simulink model "explicitCompFilter_uORB"  (R2024b)
settings: Solver=FixedStepAuto  StartTime=0.0  StopTime=35  FixedStep=0.005  RelTol=1e-3  EnableMultiTasking=on
PreLoadFcn:
  | %b_prev = Simulink.Signal;
  | %q_prev = Simulink.Signal;
  | 
  | %b_prev.InitialValue = '[0; 0; 0]';
  | %q_prev.InitialValue = '[0; 0; 0; 0]';
InitFcn:
  | %g_or = [0;0;-9.81];
  | %m_or = [27.5550; 2.4169; 16.0849];
  | gyroBias = [1; 1; 0.5];
  | 
  | %IF USING BUILT-IN UAV ANIMATION, uncomment below
  | 
  | %CLEAR UAV ANIMATIONS
  | %figHandles = findall(groot, 'Type', 'figure');
  | 
  | %for i=1:size(figHandles)
  | %    figObj = figHandles(i);
  | %    figName = figObj.Name;
  | %   if contains(figName, 'UAV Animation');
  | %        delete(figObj);
  | %    end
  | %end
undefined symbols (not defined in the file): g
libraries: robotcorelib x3, simulink_extras x3, px4Sensorslib x2, simulink x1, matrix_library x1, vrlib x1, px4uORBlib x1
(part 2 of 3)

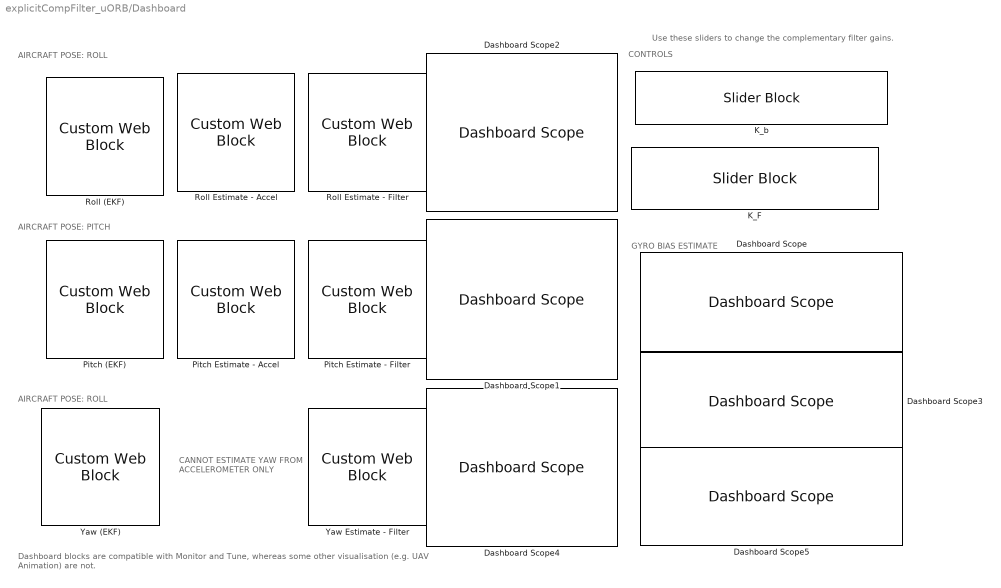
== system explicitCompFilter_uORB/Dashboard ==
  note: Dashboard blocks are compatible with Monitor and Tune, whereas some other visualisation (e.g. UAV Animation) are not.
  note: Use these sliders to change the complementary filter gains.
  note: GYRO BIAS ESTIMATE
  note: CANNOT ESTIMATE YAW
      | FROM ACCELEROMETER
      | ONLY
  note: AIRCRAFT POSE: ROLL
  note: CONTROLS
  note: AIRCRAFT POSE: PITCH
  note: AIRCRAFT POSE: ROLL
  Dashboard Scope : DashboardScope
  Dashboard Scope1 : DashboardScope  TimeSpan=10  Ymin=-10  Ymax=10  UpdateMode=Scroll  NormalizeYAxis=on
  Dashboard Scope2 : DashboardScope  TimeSpan=5  Ymin=-10  Ymax=10  UpdateMode=Scroll  NormalizeYAxis=on
  Dashboard Scope3 : DashboardScope
  Dashboard Scope4 : DashboardScope  TimeSpan=5  Ymin=-10  Ymax=10  UpdateMode=Scroll  NormalizeYAxis=on
  Dashboard Scope5 : DashboardScope
  K_F : SliderBlock  ScaleMax=10
  K_b : SliderBlock  ScaleMax=0.1  TickInterval=0.01
  Pitch (EKF) : CustomWebBlock  LabelPosition=Hide  ShowInitialText=on  Configuration="{\"components\":[{\"name\":\"CircularScaleComponent\",\"settings\":{\"bounds\":{\"max\":180,\"min\":-180,\"tickInterval\":30},\"direction\":\"cw\",\"flipLimits\":0,\"innerRadius\":0.93,\"internalTickHeightScaleFactor\":1.2,\"labelColor\":[255,255,200],\"labelFont\":{\"font\":\"Arial\",\"fontSize\":12},\"labelRadius\":0.528,\"labelTransparency\":1,\"minorTickHeightScaleFactor\":0.2,\"needleImage\":{\"size\":[967,758],\"src\":\"data:image\\/png;base64,iVBORw0KGgoAAAANSUhEUgAAA8cAAAL2CAYAAABsXuTmAAAAAXNSR0IArs4c6QAAAARnQU1BAACxjwv8YQUAAAAJcEhZcwAAMsAAADLAAShkWtsAAN3xSURBVHhe7H0HuBxXdf8akHbnnnLvzL6nbklWlyzJ6r1L7jYQg6kJHUILJXT4JyYESCAJgRA6BgKhBEwnlNgUB5tmgwGbFmyKAfduy5JV3vy\\/c+\\/c3dnZfbKe6tPT+X3f75vd2dndKbf97jn3nFpNoVAoFAqFQqFQKBQKhUKhUCgUCoVCoVAoFAqFQqFQKBQKhUKhUCgUCoVCoVAoFAqFQqFQKBQKhUKhUCgUCoVCoVAoFAqFQqFQKBQKhUKhUCgUCoVCoVAoFAqFQqFQKBQKhUKh ...(+78246 chars)\"},\"needleOffset\":[0.19,0],\"needleOrientation\":-45,\"needleRotation\":270,\"needleSize\":{\"height\":0.549,\"width\":0.7},\"outerRadius\":1,\"position\":[-0.0024794161676646707,0.022314745508982037,0.9463416916167665,1.0271800149700598],\"referencePoint\":\"auto\",\"scaleAngle\":360,\"scaleAngleOffset\":270,\"scaleColors\":[],\"scaleColorsSize\":0.2,\"scaleDirection\":\"CW\",\"scalePosition\":[0,0,1,1],\"showLabels\":false,\"showMinorTicks\":1,\"showSpanLine\":false,\"showTicks\":true,\"tickColor\":[0,0,0],\"tickTransparency\":1,\"valueBarColor\":[0,0,0],\"valueBarPosition\":[0,0,1,1],\"valueBarSize\":0.2,\"valueBarTransparency\":0}},{\"name\":\"BackgroundImageComponent\",\"settings\":{\"image\":{\"size\":[0,0],\"src\":\"default\",\"srcOrientation\":\"Right\"},\"position\":[0,0,1,1],\"scaleMode\":\"0\"}},{\"name\":\"ForegroundImageComponent\",\"settings\":{\"image\":{\"size\":[0,0],\"src\":\"default\",\"srcOrientation\":[]},\"isForeground\":1,\"position\":[0,0,1,1],\"scaleMode\":\"0\"}}],\"settings\":{\"BindingType\":\"signal\",\"aspectRatio\":1.032258064516129,\"backgroundColor\":[0,0,0,\"1\"],\"backgroundOffset\":1,\"backgroundOpacity\":1,\"direction\":\"cw\",\"fixedAspectRatio\":\"on\",\"flipLimits\":0,\"orientation\":\"horizontal\",\"showBackgroundColor\":false,\"value\":0,\"version\":\"R2023a\"},\"type\":\"CircularGauge\"}"  CustomBackgroundColor="{\"color\":[0.9019607843137255,0.9019607843137255,0.9019607843137255],\"show\":true}"
  Pitch Estimate - Accel : CustomWebBlock  LabelPosition=Hide  ShowInitialText=on  Configuration="{\"components\":[{\"name\":\"CircularScaleComponent\",\"settings\":{\"bounds\":{\"max\":180,\"min\":-180,\"tickInterval\":30},\"direction\":\"cw\",\"flipLimits\":0,\"innerRadius\":0.93,\"internalTickHeightScaleFactor\":1.2,\"labelColor\":[255,255,200],\"labelFont\":{\"font\":\"Arial\",\"fontSize\":12},\"labelRadius\":0.528,\"labelTransparency\":1,\"minorTickHeightScaleFactor\":0.2,\"needleImage\":{\"size\":[967,758],\"src\":\"data:image\\/png;base64,iVBORw0KGgoAAAANSUhEUgAAA8cAAAL2CAYAAABsXuTmAAAAAXNSR0IArs4c6QAAAARnQU1BAACxjwv8YQUAAAAJcEhZcwAAMsAAADLAAShkWtsAAN3xSURBVHhe7H0HuBxXdf8akHbnnnLvzL6nbklWlyzJ6r1L7jYQg6kJHUILJXT4JyYESCAJgRA6BgKhBEwnlNgUB5tmgwGbFmyKAfduy5JV3vy\\/c+\\/c3dnZfbKe6tPT+X3f75vd2dndKbf97jn3nFpNoVAoFAqFQqFQKBQKhUKhUCgUCoVCoVAoFAqFQqFQKBQKhUKhUCgUCoVCoVAoFAqFQqFQKBQKhUKhUCgUCoVCoVAoFAqFQqFQKBQKhUKhUCgUCoVCoVAoFAqFQqFQKBQKhUKh ...(+78246 chars)\"},\"needleOffset\":[0.19,0],\"needleOrientation\":-45,\"needleRotation\":270,\"needleSize\":{\"height\":0.549,\"width\":0.7},\"outerRadius\":1,\"position\":[-0.0024794161676646707,0.022314745508982037,0.9463416916167665,1.0271800149700598],\"referencePoint\":\"auto\",\"scaleAngle\":360,\"scaleAngleOffset\":270,\"scaleColors\":[],\"scaleColorsSize\":0.2,\"scaleDirection\":\"CW\",\"scalePosition\":[0,0,1,1],\"showLabels\":false,\"showMinorTicks\":1,\"showSpanLine\":false,\"showTicks\":true,\"tickColor\":[0,0,0],\"tickTransparency\":1,\"valueBarColor\":[0,0,0],\"valueBarPosition\":[0,0,1,1],\"valueBarSize\":0.2,\"valueBarTransparency\":0}},{\"name\":\"BackgroundImageComponent\",\"settings\":{\"image\":{\"size\":[0,0],\"src\":\"default\",\"srcOrientation\":\"Right\"},\"position\":[0,0,1,1],\"scaleMode\":\"0\"}},{\"name\":\"ForegroundImageComponent\",\"settings\":{\"image\":{\"size\":[0,0],\"src\":\"default\",\"srcOrientation\":[]},\"isForeground\":1,\"position\":[0,0,1,1],\"scaleMode\":\"0\"}}],\"settings\":{\"BindingType\":\"signal\",\"aspectRatio\":1.032258064516129,\"backgroundColor\":[0,0,0,\"1\"],\"backgroundOffset\":1,\"backgroundOpacity\":1,\"direction\":\"cw\",\"fixedAspectRatio\":\"on\",\"flipLimits\":0,\"orientation\":\"horizontal\",\"showBackgroundColor\":false,\"value\":0,\"version\":\"R2023a\"},\"type\":\"CircularGauge\"}"  CustomBackgroundColor="{\"color\":[0.9019607843137255,0.9019607843137255,0.9019607843137255],\"show\":true}"
  Pitch Estimate - Filter : CustomWebBlock  LabelPosition=Hide  ShowInitialText=on  Configuration="{\"components\":[{\"name\":\"CircularScaleComponent\",\"settings\":{\"bounds\":{\"max\":180,\"min\":-180,\"tickInterval\":30},\"direction\":\"cw\",\"flipLimits\":0,\"innerRadius\":0.93,\"internalTickHeightScaleFactor\":1.2,\"labelColor\":[255,255,200],\"labelFont\":{\"font\":\"Arial\",\"fontSize\":12},\"labelRadius\":0.528,\"labelTransparency\":1,\"minorTickHeightScaleFactor\":0.2,\"needleImage\":{\"size\":[967,758],\"src\":\"data:image\\/png;base64,iVBORw0KGgoAAAANSUhEUgAAA8cAAAL2CAYAAABsXuTmAAAAAXNSR0IArs4c6QAAAARnQU1BAACxjwv8YQUAAAAJcEhZcwAAMsAAADLAAShkWtsAAN3xSURBVHhe7H0HuBxXdf8akHbnnnLvzL6nbklWlyzJ6r1L7jYQg6kJHUILJXT4JyYESCAJgRA6BgKhBEwnlNgUB5tmgwGbFmyKAfduy5JV3vy\\/c+\\/c3dnZfbKe6tPT+X3f75vd2dndKbf97jn3nFpNoVAoFAqFQqFQKBQKhUKhUCgUCoVCoVAoFAqFQqFQKBQKhUKhUCgUCoVCoVAoFAqFQqFQKBQKhUKhUCgUCoVCoVAoFAqFQqFQKBQKhUKhUCgUCoVCoVAoFAqFQqFQKBQKhUKh ...(+78246 chars)\"},\"needleOffset\":[0.19,0],\"needleOrientation\":-45,\"needleRotation\":270,\"needleSize\":{\"height\":0.549,\"width\":0.7},\"outerRadius\":1,\"position\":[-0.0024794161676646707,0.022314745508982037,0.9463416916167665,1.0271800149700598],\"referencePoint\":\"auto\",\"scaleAngle\":360,\"scaleAngleOffset\":270,\"scaleColors\":[],\"scaleColorsSize\":0.2,\"scaleDirection\":\"CW\",\"scalePosition\":[0,0,1,1],\"showLabels\":false,\"showMinorTicks\":1,\"showSpanLine\":false,\"showTicks\":true,\"tickColor\":[0,0,0],\"tickTransparency\":1,\"valueBarColor\":[0,0,0],\"valueBarPosition\":[0,0,1,1],\"valueBarSize\":0.2,\"valueBarTransparency\":0}},{\"name\":\"BackgroundImageComponent\",\"settings\":{\"image\":{\"size\":[0,0],\"src\":\"default\",\"srcOrientation\":\"Right\"},\"position\":[0,0,1,1],\"scaleMode\":\"0\"}},{\"name\":\"ForegroundImageComponent\",\"settings\":{\"image\":{\"size\":[0,0],\"src\":\"default\",\"srcOrientation\":[]},\"isForeground\":1,\"position\":[0,0,1,1],\"scaleMode\":\"0\"}}],\"settings\":{\"BindingType\":\"signal\",\"aspectRatio\":1.032258064516129,\"backgroundColor\":[0,0,0,\"1\"],\"backgroundOffset\":1,\"backgroundOpacity\":1,\"direction\":\"cw\",\"fixedAspectRatio\":\"on\",\"flipLimits\":0,\"orientation\":\"horizontal\",\"showBackgroundColor\":false,\"value\":0,\"version\":\"R2023a\"},\"type\":\"CircularGauge\"}"  CustomBackgroundColor="{\"color\":[0.9019607843137255,0.9019607843137255,0.9019607843137255],\"show\":true}"
  Roll (EKF) : CustomWebBlock  LabelPosition=Hide  ShowInitialText=on  Configuration="{\"components\":[{\"name\":\"CircularScaleComponent\",\"settings\":{\"bounds\":{\"max\":180,\"min\":-180,\"tickInterval\":30},\"direction\":\"cw\",\"flipLimits\":0,\"innerRadius\":0.93,\"internalTickHeightScaleFactor\":1.2,\"labelColor\":[255,255,200],\"labelFont\":{\"font\":\"Arial\",\"fontSize\":12},\"labelRadius\":0.528,\"labelTransparency\":1,\"minorTickHeightScaleFactor\":0.2,\"needleImage\":{\"size\":[967,835],\"src\":\"data:image\\/png;base64,iVBORw0KGgoAAAANSUhEUgAAA8cAAANDCAYAAACALm2UAAAAAXNSR0IArs4c6QAAAARnQU1BAACxjwv8YQUAAAAJcEhZcwAAMsAAADLAAShkWtsAANscSURBVHhe7J0HnBxHlf\\/XxtZOV733qnpmg6Jl5WBZVrCsnGU5YZPjwQEHR4Y\\/4Q6OcHB3wN0R7shHMjma5OPIxmBycCAYAwYMNhgHnIMsWWn7\\/3nVXTM9PbvSSlba1e\\/7+fx2Znt6Znq6q6vqVb16r6sLAAAAAAAAAAAAAAAAAAAAAAAAAAAAAAAAAAAAAAAAAAAAAAAAAAAAAAAAAAAAAAAAAAAAAAAAAAAAAAAAAAAAAAAAAAAAAAAAAAAAAAAAAAAAAAAAAAAAAAAAAAAA ...(+77442 chars)\"},\"needleOffset\":[0.16,0],\"needleOrientation\":-45,\"needleRotation\":270,\"needleSize\":{\"height\":0.604,\"width\":0.7},\"outerRadius\":1,\"position\":[-0.0024794161676646707,0.022314745508982037,0.9463416916167665,1.0271800149700598],\"referencePoint\":\"auto\",\"scaleAngle\":360,\"scaleAngleOffset\":270,\"scaleColors\":[],\"scaleColorsSize\":0.2,\"scaleDirection\":\"CCW\",\"scalePosition\":[0,0,1,1],\"showLabels\":false,\"showMinorTicks\":1,\"showSpanLine\":false,\"showTicks\":true,\"tickColor\":[0,0,0],\"tickTransparency\":1,\"valueBarColor\":[0,0,0],\"valueBarPosition\":[0,0,1,1],\"valueBarSize\":0.2,\"valueBarTransparency\":0}},{\"name\":\"BackgroundImageComponent\",\"settings\":{\"image\":{\"size\":[0,0],\"src\":\"default\",\"srcOrientation\":\"Right\"},\"position\":[0,0,1,1],\"scaleMode\":\"0\"}},{\"name\":\"ForegroundImageComponent\",\"settings\":{\"image\":{\"size\":[0,0],\"src\":\"default\",\"srcOrientation\":[]},\"isForeground\":1,\"position\":[0,0,1,1],\"scaleMode\":\"0\"}}],\"settings\":{\"BindingType\":\"signal\",\"aspectRatio\":1.032258064516129,\"backgroundColor\":[0,0,0,\"1\"],\"backgroundOffset\":1,\"backgroundOpacity\":1,\"direction\":\"cw\",\"fixedAspectRatio\":\"on\",\"flipLimits\":0,\"orientation\":\"horizontal\",\"showBackgroundColor\":false,\"value\":0,\"version\":\"R2023a\"},\"type\":\"CircularGauge\"}"  CustomBackgroundColor="{\"color\":[0.9019607843137255,0.9019607843137255,0.9019607843137255],\"show\":true}"
  Roll Estimate - Accel : CustomWebBlock  LabelPosition=Hide  ShowInitialText=on  Configuration="{\"components\":[{\"name\":\"CircularScaleComponent\",\"settings\":{\"bounds\":{\"max\":180,\"min\":-180,\"tickInterval\":30},\"direction\":\"cw\",\"flipLimits\":0,\"innerRadius\":0.93,\"internalTickHeightScaleFactor\":1.2,\"labelColor\":[255,255,200],\"labelFont\":{\"font\":\"Arial\",\"fontSize\":12},\"labelRadius\":0.528,\"labelTransparency\":1,\"minorTickHeightScaleFactor\":0.2,\"needleImage\":{\"size\":[967,835],\"src\":\"data:image\\/png;base64,iVBORw0KGgoAAAANSUhEUgAAA8cAAANDCAYAAACALm2UAAAAAXNSR0IArs4c6QAAAARnQU1BAACxjwv8YQUAAAAJcEhZcwAAMsAAADLAAShkWtsAANscSURBVHhe7J0HnBxHlf\\/XxtZOV733qnpmg6Jl5WBZVrCsnGU5YZPjwQEHR4Y\\/4Q6OcHB3wN0R7shHMjma5OPIxmBycCAYAwYMNhgHnIMsWWn7\\/3nVXTM9PbvSSlba1e\\/7+fx2Znt6Znq6q6vqVb16r6sLAAAAAAAAAAAAAAAAAAAAAAAAAAAAAAAAAAAAAAAAAAAAAAAAAAAAAAAAAAAAAAAAAAAAAAAAAAAAAAAAAAAAAAAAAAAAAAAAAAAAAAAAAAAAAAAAAAAAAAAAAAAA ...(+77442 chars)\"},\"needleOffset\":[0.16,0],\"needleOrientation\":-45,\"needleRotation\":270,\"needleSize\":{\"height\":0.604,\"width\":0.7},\"outerRadius\":1,\"position\":[-0.0024794161676646707,0.022314745508982037,0.9463416916167665,1.0271800149700598],\"referencePoint\":\"auto\",\"scaleAngle\":360,\"scaleAngleOffset\":270,\"scaleColors\":[],\"scaleColorsSize\":0.2,\"scaleDirection\":\"CCW\",\"scalePosition\":[0,0,1,1],\"showLabels\":false,\"showMinorTicks\":1,\"showSpanLine\":false,\"showTicks\":true,\"tickColor\":[0,0,0],\"tickTransparency\":1,\"valueBarColor\":[0,0,0],\"valueBarPosition\":[0,0,1,1],\"valueBarSize\":0.2,\"valueBarTransparency\":0}},{\"name\":\"BackgroundImageComponent\",\"settings\":{\"image\":{\"size\":[0,0],\"src\":\"default\",\"srcOrientation\":\"Right\"},\"position\":[0,0,1,1],\"scaleMode\":\"0\"}},{\"name\":\"ForegroundImageComponent\",\"settings\":{\"image\":{\"size\":[0,0],\"src\":\"default\",\"srcOrientation\":[]},\"isForeground\":1,\"position\":[0,0,1,1],\"scaleMode\":\"0\"}}],\"settings\":{\"BindingType\":\"signal\",\"aspectRatio\":1.032258064516129,\"backgroundColor\":[0,0,0,\"1\"],\"backgroundOffset\":1,\"backgroundOpacity\":1,\"direction\":\"cw\",\"fixedAspectRatio\":\"on\",\"flipLimits\":0,\"orientation\":\"horizontal\",\"showBackgroundColor\":false,\"value\":0,\"version\":\"R2023a\"},\"type\":\"CircularGauge\"}"  CustomBackgroundColor="{\"color\":[0.9019607843137255,0.9019607843137255,0.9019607843137255],\"show\":true}"
  Roll Estimate - Filter : CustomWebBlock  LabelPosition=Hide  ShowInitialText=on  Configuration="{\"components\":[{\"name\":\"CircularScaleComponent\",\"settings\":{\"bounds\":{\"max\":180,\"min\":-180,\"tickInterval\":30},\"direction\":\"cw\",\"flipLimits\":0,\"innerRadius\":0.93,\"internalTickHeightScaleFactor\":1.2,\"labelColor\":[255,255,200],\"labelFont\":{\"font\":\"Arial\",\"fontSize\":12},\"labelRadius\":0.528,\"labelTransparency\":1,\"minorTickHeightScaleFactor\":0.2,\"needleImage\":{\"size\":[967,835],\"src\":\"data:image\\/png;base64,iVBORw0KGgoAAAANSUhEUgAAA8cAAANDCAYAAACALm2UAAAAAXNSR0IArs4c6QAAAARnQU1BAACxjwv8YQUAAAAJcEhZcwAAMsAAADLAAShkWtsAANscSURBVHhe7J0HnBxHlf\\/XxtZOV733qnpmg6Jl5WBZVrCsnGU5YZPjwQEHR4Y\\/4Q6OcHB3wN0R7shHMjma5OPIxmBycCAYAwYMNhgHnIMsWWn7\\/3nVXTM9PbvSSlba1e\\/7+fx2Znt6Znq6q6vqVb16r6sLAAAAAAAAAAAAAAAAAAAAAAAAAAAAAAAAAAAAAAAAAAAAAAAAAAAAAAAAAAAAAAAAAAAAAAAAAAAAAAAAAAAAAAAAAAAAAAAAAAAAAAAAAAAAAAAAAAAAAAAAAAAA ...(+77442 chars)\"},\"needleOffset\":[0.16,0],\"needleOrientation\":-45,\"needleRotation\":270,\"needleSize\":{\"height\":0.604,\"width\":0.7},\"outerRadius\":1,\"position\":[-0.0024794161676646707,0.022314745508982037,0.9463416916167665,1.0271800149700598],\"referencePoint\":\"auto\",\"scaleAngle\":360,\"scaleAngleOffset\":270,\"scaleColors\":[],\"scaleColorsSize\":0.2,\"scaleDirection\":\"CCW\",\"scalePosition\":[0,0,1,1],\"showLabels\":false,\"showMinorTicks\":1,\"showSpanLine\":false,\"showTicks\":true,\"tickColor\":[0,0,0],\"tickTransparency\":1,\"valueBarColor\":[0,0,0],\"valueBarPosition\":[0,0,1,1],\"valueBarSize\":0.2,\"valueBarTransparency\":0}},{\"name\":\"BackgroundImageComponent\",\"settings\":{\"image\":{\"size\":[0,0],\"src\":\"default\",\"srcOrientation\":\"Right\"},\"position\":[0,0,1,1],\"scaleMode\":\"0\"}},{\"name\":\"ForegroundImageComponent\",\"settings\":{\"image\":{\"size\":[0,0],\"src\":\"default\",\"srcOrientation\":[]},\"isForeground\":1,\"position\":[0,0,1,1],\"scaleMode\":\"0\"}}],\"settings\":{\"BindingType\":\"signal\",\"aspectRatio\":1.032258064516129,\"backgroundColor\":[0,0,0,\"1\"],\"backgroundOffset\":1,\"backgroundOpacity\":1,\"direction\":\"cw\",\"fixedAspectRatio\":\"on\",\"flipLimits\":0,\"orientation\":\"horizontal\",\"showBackgroundColor\":false,\"value\":0,\"version\":\"R2023a\"},\"type\":\"CircularGauge\"}"  CustomBackgroundColor="{\"color\":[0.9019607843137255,0.9019607843137255,0.9019607843137255],\"show\":true}"
  Yaw (EKF) : CustomWebBlock  LabelPosition=Hide  ShowInitialText=on  Configuration="{\"components\":[{\"name\":\"CircularScaleComponent\",\"settings\":{\"bounds\":{\"max\":180,\"min\":-180,\"tickInterval\":30},\"direction\":\"cw\",\"flipLimits\":0,\"innerRadius\":0.93,\"internalTickHeightScaleFactor\":1.2,\"labelColor\":[255,255,200],\"labelFont\":{\"font\":\"Arial\",\"fontSize\":12},\"labelRadius\":0.528,\"labelTransparency\":1,\"minorTickHeightScaleFactor\":0.2,\"needleImage\":{\"size\":[277,410],\"src\":\"data:image\\/png;base64,iVBORw0KGgoAAAANSUhEUgAAARUAAAGaCAYAAAAhCNfvAAAAAXNSR0IArs4c6QAAAARnQU1BAACxjwv8YQUAAAAJcEhZcwAAFxEAABcRAcom8z8AACNWSURBVHhe7Z0J3H\\/ZXMe\\/zxTJMoYsSTGWRCRLCS0UlVT2ZEkREqNIFG1KRAuTkoSMIsnSCCVL\\/WfsicgIUWas2Se7Nnq9Z85v5pnzv8\\/z\\/O493\\/t77u\\/e9\\/v1+rzMjN9z7+937jmfe873nPM9ESIiIiIiIiIiIiIiIiIiIiIiIiIiIiIiIiIiIiIiIiIiIiIiIiIiIiIiIiIiIiIiIiIiIiIiIiIiIiIyQc4fEVeKiJtGxE9ExH0j4j4R8W0R8aX1hyUuGhHXiYgb ...(+12100 chars)\"},\"needleOffset\":[0.1,0],\"needleOrientation\":-45,\"needleRotation\":270,\"needleSize\":{\"height\":0.6,\"width\":0.405},\"outerRadius\":1,\"position\":[-0.0024794161676646707,0.022314745508982037,0.9463416916167665,1.0271800149700598],\"referencePoint\":\"auto\",\"scaleAngle\":360,\"scaleAngleOffset\":90,\"scaleColors\":[],\"scaleColorsSize\":0.2,\"scaleDirection\":\"CW\",\"scalePosition\":[0,0,1,1],\"showLabels\":false,\"showMinorTicks\":1,\"showSpanLine\":false,\"showTicks\":true,\"tickColor\":[0,0,0],\"tickTransparency\":1,\"valueBarColor\":[0,0,0],\"valueBarPosition\":[0,0,1,1],\"valueBarSize\":0.2,\"valueBarTransparency\":0}},{\"name\":\"BackgroundImageComponent\",\"settings\":{\"image\":{\"size\":[0,0],\"src\":\"default\",\"srcOrientation\":\"Right\"},\"position\":[0,0,1,1],\"scaleMode\":\"0\"}},{\"name\":\"ForegroundImageComponent\",\"settings\":{\"image\":{\"size\":[0,0],\"src\":\"default\",\"srcOrientation\":[]},\"isForeground\":1,\"position\":[0,0,1,1],\"scaleMode\":\"0\"}}],\"settings\":{\"BindingType\":\"signal\",\"aspectRatio\":1.032258064516129,\"backgroundColor\":[0,0,0,\"1\"],\"backgroundOffset\":1,\"backgroundOpacity\":1,\"direction\":\"cw\",\"fixedAspectRatio\":\"on\",\"flipLimits\":0,\"orientation\":\"horizontal\",\"showBackgroundColor\":false,\"value\":0,\"version\":\"R2023a\"},\"type\":\"CircularGauge\"}"  CustomBackgroundColor="{\"color\":[0.9019607843137255,0.9019607843137255,0.9019607843137255],\"show\":true}"
  Yaw Estimate - Filter : CustomWebBlock  LabelPosition=Hide  ShowInitialText=on  Configuration="{\"components\":[{\"name\":\"CircularScaleComponent\",\"settings\":{\"bounds\":{\"max\":180,\"min\":-180,\"tickInterval\":30},\"direction\":\"cw\",\"flipLimits\":0,\"innerRadius\":0.93,\"internalTickHeightScaleFactor\":1.2,\"labelColor\":[255,255,200],\"labelFont\":{\"font\":\"Arial\",\"fontSize\":12},\"labelRadius\":0.528,\"labelTransparency\":1,\"minorTickHeightScaleFactor\":0.2,\"needleImage\":{\"size\":[277,410],\"src\":\"data:image\\/png;base64,iVBORw0KGgoAAAANSUhEUgAAARUAAAGaCAYAAAAhCNfvAAAAAXNSR0IArs4c6QAAAARnQU1BAACxjwv8YQUAAAAJcEhZcwAAFxEAABcRAcom8z8AACNWSURBVHhe7Z0J3H\\/ZXMe\\/zxTJMoYsSTGWRCRLCS0UlVT2ZEkREqNIFG1KRAuTkoSMIsnSCCVL\\/WfsicgIUWas2Se7Nnq9Z85v5pnzv8\\/z\\/O493\\/t77u\\/e9\\/v1+rzMjN9z7+937jmfe873nPM9ESIiIiIiIiIiIiIiIiIiIiIiIiIiIiIiIiIiIiIiIiIiIiIiIiIiIiIiIiIiIiIiIiIiIiIiIiIiIiIyQc4fEVeKiJtGxE9ExH0j4j4R8W0R8aX1hyUuGhHXiYgb ...(+12100 chars)\"},\"needleOffset\":[0.1,0],\"needleOrientation\":-45,\"needleRotation\":270,\"needleSize\":{\"height\":0.6,\"width\":0.405},\"outerRadius\":1,\"position\":[-0.010096153846153847,0.022235576923076924,0.9462740384615385,1.0271634615384615],\"referencePoint\":\"auto\",\"scaleAngle\":360,\"scaleAngleOffset\":90,\"scaleColors\":[],\"scaleColorsSize\":0.2,\"scaleDirection\":\"CW\",\"scalePosition\":[0,0,1,1],\"showLabels\":false,\"showMinorTicks\":1,\"showSpanLine\":false,\"showTicks\":true,\"tickColor\":[0,0,0],\"tickTransparency\":1,\"valueBarColor\":[0,0,0],\"valueBarPosition\":[0,0,1,1],\"valueBarSize\":0.2,\"valueBarTransparency\":0}},{\"name\":\"BackgroundImageComponent\",\"settings\":{\"image\":{\"size\":[0,0],\"src\":\"default\",\"srcOrientation\":\"Right\"},\"position\":[0,0,1,1],\"scaleMode\":\"0\"}},{\"name\":\"ForegroundImageComponent\",\"settings\":{\"image\":{\"size\":[0,0],\"src\":\"default\",\"srcOrientation\":[]},\"isForeground\":1,\"position\":[0,0,1,1],\"scaleMode\":\"0\"}}],\"settings\":{\"BindingType\":\"signal\",\"aspectRatio\":1.032258064516129,\"backgroundColor\":[0,0,0,\"1\"],\"backgroundOffset\":1,\"backgroundOpacity\":1,\"direction\":\"cw\",\"fixedAspectRatio\":\"on\",\"flipLimits\":0,\"orientation\":\"horizontal\",\"showBackgroundColor\":false,\"value\":0,\"version\":\"R2023a\"},\"type\":\"CircularGauge\"}"  CustomBackgroundColor="{\"color\":[0.9019607843137255,0.9019607843137255,0.9019607843137255],\"show\":true}"
